simulink library "Aerodynamics_lib"  (R2020a)
settings: Solver=VariableStepAuto  StartTime=0.0  StopTime=10.0  RelTol=1e-3
undefined symbols (not defined in the file or in its folder): bref, CD0, CD_alpha, CL0, Cl_aileron, CL_alpha, CL_alphadot, Cl_beta, CL_elev, Cl_p, CL_q, Cl_r, Cl_rudder, Cm0, Cm_alpha, Cm_alphadot, Cm_elev, Cm_q, Cn_aileron, Cn_beta, Cn_p, Cn_r, Cn_rudder, cref, CY_beta, CY_p, CY_r, CY_rudder, Sref, X_CG, Z_CG
settings Model: Creator=muril  LastModifiedBy=muril

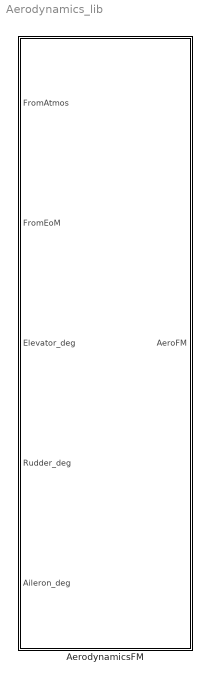
== system Aerodynamics_lib ==
  AerodynamicsFM : Subsystem

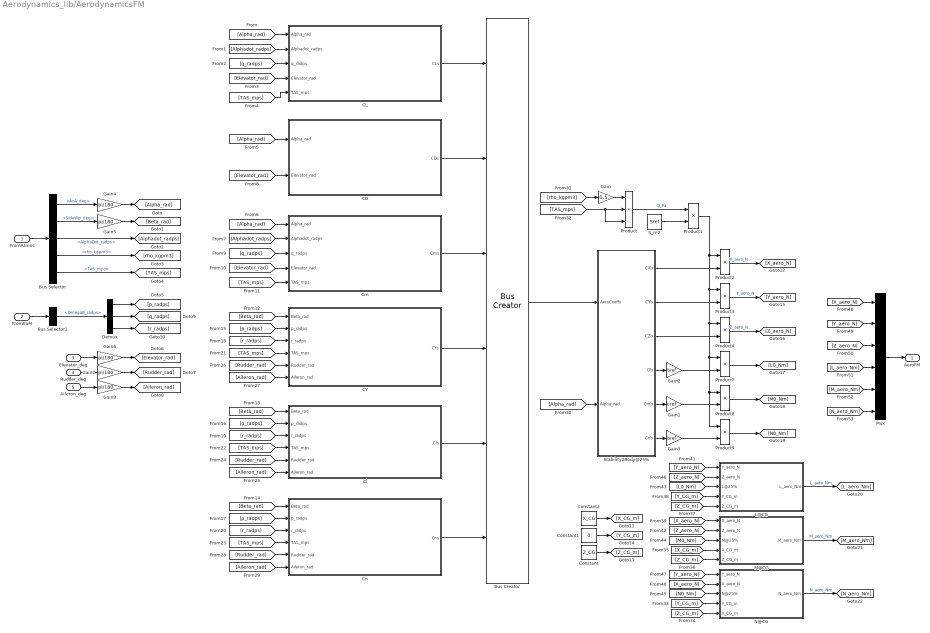
== system Aerodynamics_lib/AerodynamicsFM ==
  FromAtmos : Inport
  FromEoM : Inport  Port=2
  Elevator_deg : Inport  Port=3
  Rudder_deg : Inport  Port=4
  Aileron_deg : Inport  Port=5
  Bus Creator : BusCreator  Inputs=6
  Bus Selector : BusSelector  OutputSignals=AoA_deg,Sideslip_deg,AlphaDot_radps,rho_kgpm3,TAS_mps
  Bus Selector1 : BusSelector  OutputSignals=OmegaB_radps
  CD : Subsystem
  CL : Subsystem
  CY : Subsystem
  Cl : Subsystem
  Cm : Subsystem
  Cn : Subsystem
  Constant : Constant  Value=Z_CG
  Constant1 : Constant  Value=0
  Constant2 : Constant  Value=X_CG
  Demux : Demux  Outputs=3
  Gain : Gain  Gain=0.5
  Gain1 : Gain  Gain=cref
  Gain2 : Gain  Gain=bref
  Gain3 : Gain  Gain=bref
  Gain{4..8} (5 alike) : Gain  Gain=pi/180
  L@CG : Subsystem
  M@CG : Subsystem
  Mux : Mux  Inputs=6
  N@CG : Subsystem
  Product : Product  Inputs=3
  Product{1..4,7..9} (7 alike) : Product
  S_m2 : Constant  Value=Sref
  Stability2Body@25% : Subsystem
  AeroFM : Outport
  wires:
  Constant2/1 -> [X_CG_m]
  Constant/1 -> [Z_CG_m]
  Bus Selector1/1 -> Demux/1  "<OmegaB_radps>"
  FromEoM/1 -> Bus Selector1/1
  Bus Selector/3 -> [Alphadot_radps]  "<AlphaDot_radps>"
  Bus Selector/2 -> Gain5/1  "<Sideslip_deg>"
  Bus Selector/1 -> Gain4/1  "<AoA_deg>"
  FromAtmos/1 -> Bus Selector/1
  [q_radps] -> CL/3(q_radps)
  [Alpha_rad] -> CL/1(Alpha_rad)
  Stability2Body@25%/2(CYb) -> Product3/2
  [Beta_rad] -> Cl/1(Beta_rad)
  Gain8/1 -> [Aileron_rad]
  Elevator_deg/1 -> Gain6/1
  Product1/1 -> Product9/1, Product8/1, Product7/1, Product4/1, Product3/1, Product2/1
  Bus Selector/5 -> [TAS_mps]  "<TAS_mps>"
  Product/1 -> Product1/1  "Q_Pa"
  [Alpha_rad] -> CD/1(Alpha_rad)
  Product8/1 -> [M0_Nm]
  Gain7/1 -> [Rudder_rad]
  Demux/1 -> [p_radps]
  [Alphadot_radps] -> CL/2(Alphadot_radps)
  [r_radps] -> Cl/3(r_radps)
  CD/1(CDs) -> Bus Creator/2
  Aileron_deg/1 -> Gain8/1
  [p_radps] -> Cl/2(p_radps)
  [TAS_mps] -> CL/5(TAS_mps)
  [Alphadot_radps] -> Cm/2(Alphadot_radps)
  [Alpha_rad] -> Cm/1(Alpha_rad)
  [TAS_mps] -> Cm/5(TAS_mps)
  [Beta_rad] -> Cn/1(Beta_rad)
  Gain6/1 -> [Elevator_rad]
  [TAS_mps] -> Product/3, Product/2
  N@CG/1(N_aero_Nm) -> [N_aero_Nm]  "N_aero_Nm"
  [Elevator_rad] -> CD/2(Elevator_rad)
  Gain5/1 -> [Beta_rad]
  Stability2Body@25%/3(CZb) -> Product4/2
  Gain3/1 -> Product9/2
  Product3/1 -> [Y_aero_N]  "Y_aero_N"
  [Aileron_rad] -> Cl/6(Aileron_rad)
  [TAS_mps] -> CY/4(TAS_mps)
  Demux/2 -> [q_radps]
  [TAS_mps] -> Cn/4(TAS_mps)
  [Rudder_rad] -> Cl/5(Rudder_rad)
  [Aileron_rad] -> Cn/6(Aileron_rad)
  [r_radps] -> Cn/3(r_radps)
  CL/1(CLs) -> Bus Creator/1
  [Beta_rad] -> CY/1(Beta_rad)
  [Z_CG_m] -> M@CG/5(Z_CG_m)
  S_m2/1 -> Product1/2
  Stability2Body@25%/4(Clb) -> Gain2/1
  [p_radps] -> CY/2(p_radps)
  Stability2Body@25%/1(CXb) -> Product2/2
  [p_radps] -> Cn/2(p_radps)
  [TAS_mps] -> Cl/4(TAS_mps)
  Gain/1 -> Product/1
  CY/1(CYs) -> Bus Creator/4
  [Rudder_rad] -> Cn/5(Rudder_rad)
  Constant1/1 -> [Y_CG_m]
  Cm/1(Cms) -> Bus Creator/3
  Gain1/1 -> Product8/2
  [Rudder_rad] -> CY/5(Rudder_rad)
  Gain2/1 -> Product7/2
  Cn/1(Cns) -> Bus Creator/6
  [Y_aero_N] -> Mux/2
  Stability2Body@25%/5(Cmb) -> Gain1/1
  [Aileron_rad] -> CY/6(Aileron_rad)
  Rudder_deg/1 -> Gain7/1
  Bus Creator/1 -> Stability2Body@25%/1(AeroCoeffs)
  Product2/1 -> [X_aero_N]  "X_aero_N"
  [X_aero_N] -> M@CG/1(X_aero_N)
  [r_radps] -> CY/3(r_radps)
  [Z_CG_m] -> L@CG/5(Z_CG_m)
  [X_CG_m] -> M@CG/4(X_CG_m)
  [Y_CG_m] -> L@CG/4(Y_CG_m)
  Bus Selector/4 -> [rho_kgpm3]  "<rho_kgpm3>"
  Cl/1(Cls) -> Bus Creator/5
  [q_radps] -> Cm/3(q_radps)
  [Elevator_rad] -> Cm/4(Elevator_rad)
  Product4/1 -> [Z_aero_N]  "Z_aero_N"
  Demux/3 -> [r_radps]
  [Alpha_rad] -> Stability2Body@25%/2(Alpha_rad)
  Product9/1 -> [N0_Nm]
  Gain4/1 -> [Alpha_rad]
  M@CG/1(M_aero_Nm) -> [M_aero_Nm]  "M_aero_Nm"
  [M0_Nm] -> M@CG/3(M@25%)
  [rho_kgpm3] -> Gain/1
  [Z_aero_N] -> L@CG/2(Z_aero_N)
  [Y_aero_N] -> L@CG/1(Y_aero_N)
  [X_aero_N] -> N@CG/2(X_aero_N)
  [Z_CG_m] -> N@CG/5(X_CG_m)
  Product7/1 -> [L0_Nm]
  Mux/1 -> AeroFM/1
  [Z_aero_N] -> Mux/3
  [L0_Nm] -> L@CG/3(L@25%)
  Stability2Body@25%/6(Cnb) -> Gain3/1
  [Y_CG_m] -> N@CG/4(Y_CG_m)
  [N0_Nm] -> N@CG/3(N@25%)
  [Elevator_rad] -> CL/4(Elevator_rad)
  [Y_aero_N] -> N@CG/1(Y_aero_N)
  [L_aero_Nm] -> Mux/4
  [X_aero_N] -> Mux/1
  [Z_aero_N] -> M@CG/2(Z_aero_N)
  [M_aero_Nm] -> Mux/5
  L@CG/1(L_aero_Nm) -> [L_aero_Nm]  "L_aero_Nm"
  [N_aero_Nm] -> Mux/6

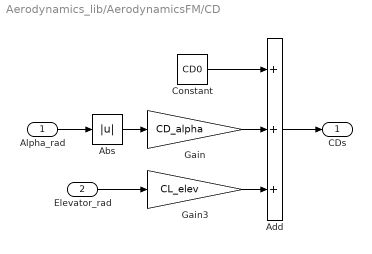
== system Aerodynamics_lib/AerodynamicsFM/CD ==
  Alpha_rad : Inport
  Elevator_rad : Inport  Port=2
  Abs : Abs
  Add : Sum  Inputs=+++
  Constant : Constant  Value=CD0
  Gain : Gain  Gain=CD_alpha
  Gain3 : Gain  Gain=CL_elev
  CDs : Outport
  wires:
  Gain3/1 -> Add/3
  Add/1 -> CDs/1
  Gain/1 -> Add/2
  Constant/1 -> Add/1
  Elevator_rad/1 -> Gain3/1
  Abs/1 -> Gain/1
  Alpha_rad/1 -> Abs/1

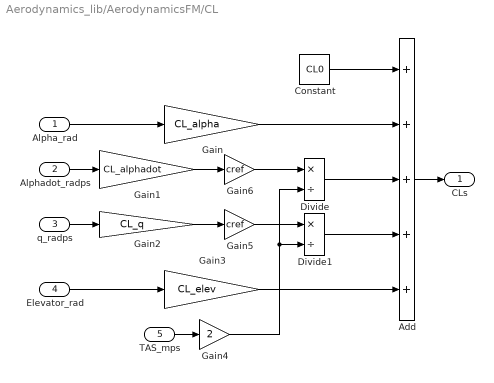
== system Aerodynamics_lib/AerodynamicsFM/CL ==
  Alpha_rad : Inport
  Alphadot_radps : Inport  Port=2
  q_radps : Inport  Port=3
  Elevator_rad : Inport  Port=4
  TAS_mps : Inport  Port=5
  Add : Sum  Inputs=+++++
  Constant : Constant  Value=CL0
  Divide : Product  Inputs=*/
  Divide1 : Product  Inputs=*/
  Gain : Gain  Gain=CL_alpha
  Gain1 : Gain  Gain=CL_alphadot
  Gain2 : Gain  Gain=CL_q
  Gain3 : Gain  Gain=CL_elev
  Gain4 : Gain  Gain=2
  Gain5 : Gain  Gain=cref
  Gain6 : Gain  Gain=cref
  CLs : Outport
  wires:
  Gain3/1 -> Add/5
  Alpha_rad/1 -> Gain/1
  Elevator_rad/1 -> Gain3/1
  Gain/1 -> Add/2
  Alphadot_radps/1 -> Gain1/1
  Constant/1 -> Add/1
  Add/1 -> CLs/1
  TAS_mps/1 -> Gain4/1
  Gain1/1 -> Gain6/1
  Gain6/1 -> Divide/1
  Gain4/1 -> Divide/2, Divide1/2
  Divide/1 -> Add/3
  Divide1/1 -> Add/4
  Gain5/1 -> Divide1/1
  Gain2/1 -> Gain5/1
  q_radps/1 -> Gain2/1

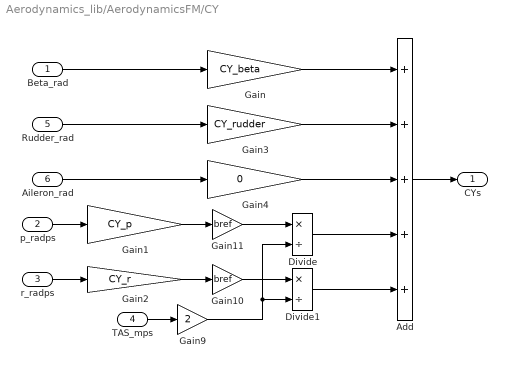
== system Aerodynamics_lib/AerodynamicsFM/CY ==
  Beta_rad : Inport
  p_radps : Inport  Port=2
  r_radps : Inport  Port=3
  TAS_mps : Inport  Port=4
  Rudder_rad : Inport  Port=5
  Aileron_rad : Inport  Port=6
  Add : Sum  Inputs=+++++
  Divide : Product  Inputs=*/
  Divide1 : Product  Inputs=*/
  Gain : Gain  Gain=CY_beta
  Gain1 : Gain  Gain=CY_p
  Gain10 : Gain  Gain=bref
  Gain11 : Gain  Gain=bref
  Gain2 : Gain  Gain=CY_r
  Gain3 : Gain  Gain=CY_rudder
  Gain4 : Gain  Gain=0
  Gain9 : Gain  Gain=2
  CYs : Outport
  wires:
  Gain9/1 -> Divide/2, Divide1/2
  p_radps/1 -> Gain1/1
  Gain1/1 -> Gain11/1
  TAS_mps/1 -> Gain9/1
  Add/1 -> CYs/1
  r_radps/1 -> Gain2/1
  Gain2/1 -> Gain10/1
  Gain10/1 -> Divide1/1
  Beta_rad/1 -> Gain/1
  Gain11/1 -> Divide/1
  Gain/1 -> Add/1
  Divide/1 -> Add/4
  Divide1/1 -> Add/5
  Rudder_rad/1 -> Gain3/1
  Aileron_rad/1 -> Gain4/1
  Gain4/1 -> Add/3
  Gain3/1 -> Add/2

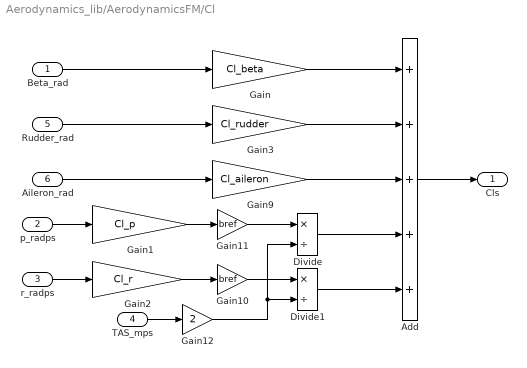
== system Aerodynamics_lib/AerodynamicsFM/Cl ==
  Beta_rad : Inport
  p_radps : Inport  Port=2
  r_radps : Inport  Port=3
  TAS_mps : Inport  Port=4
  Rudder_rad : Inport  Port=5
  Aileron_rad : Inport  Port=6
  Add : Sum  Inputs=+++++
  Divide : Product  Inputs=*/
  Divide1 : Product  Inputs=*/
  Gain : Gain  Gain=Cl_beta
  Gain1 : Gain  Gain=Cl_p
  Gain10 : Gain  Gain=bref
  Gain11 : Gain  Gain=bref
  Gain12 : Gain  Gain=2
  Gain2 : Gain  Gain=Cl_r
  Gain3 : Gain  Gain=Cl_rudder
  Gain9 : Gain  Gain=Cl_aileron
  Cls : Outport
  wires:
  r_radps/1 -> Gain2/1
  Gain12/1 -> Divide/2, Divide1/2
  Divide/1 -> Add/4
  Gain1/1 -> Gain11/1
  Gain/1 -> Add/1
  Aileron_rad/1 -> Gain9/1
  Gain10/1 -> Divide1/1
  p_radps/1 -> Gain1/1
  Divide1/1 -> Add/5
  Add/1 -> Cls/1
  TAS_mps/1 -> Gain12/1
  Gain2/1 -> Gain10/1
  Gain11/1 -> Divide/1
  Rudder_rad/1 -> Gain3/1
  Beta_rad/1 -> Gain/1
  Gain9/1 -> Add/3
  Gain3/1 -> Add/2

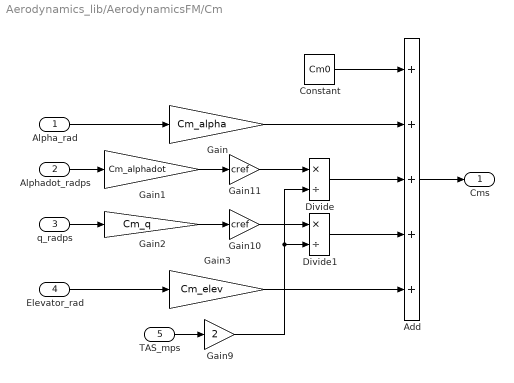
== system Aerodynamics_lib/AerodynamicsFM/Cm ==
  Alpha_rad : Inport
  Alphadot_radps : Inport  Port=2
  q_radps : Inport  Port=3
  Elevator_rad : Inport  Port=4
  TAS_mps : Inport  Port=5
  Add : Sum  Inputs=+++++
  Constant : Constant  Value=Cm0
  Divide : Product  Inputs=*/
  Divide1 : Product  Inputs=*/
  Gain : Gain  Gain=Cm_alpha
  Gain1 : Gain  Gain=Cm_alphadot
  Gain10 : Gain  Gain=cref
  Gain11 : Gain  Gain=cref
  Gain2 : Gain  Gain=Cm_q
  Gain3 : Gain  Gain=Cm_elev
  Gain9 : Gain  Gain=2
  Cms : Outport
  wires:
  Gain2/1 -> Gain10/1
  Gain/1 -> Add/2
  Gain11/1 -> Divide/1
  Gain9/1 -> Divide/2, Divide1/2
  TAS_mps/1 -> Gain9/1
  Constant/1 -> Add/1
  Divide1/1 -> Add/4
  q_radps/1 -> Gain2/1
  Gain3/1 -> Add/5
  Elevator_rad/1 -> Gain3/1
  Gain1/1 -> Gain11/1
  Alphadot_radps/1 -> Gain1/1
  Gain10/1 -> Divide1/1
  Divide/1 -> Add/3
  Alpha_rad/1 -> Gain/1
  Add/1 -> Cms/1

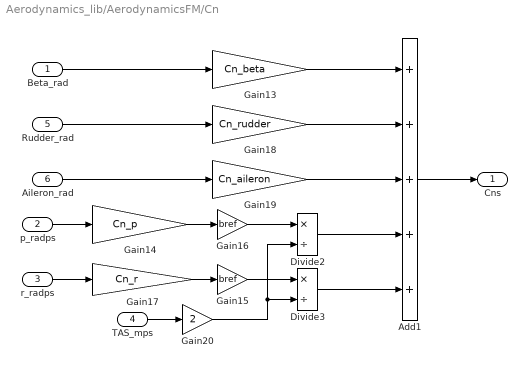
== system Aerodynamics_lib/AerodynamicsFM/Cn ==
  Beta_rad : Inport
  p_radps : Inport  Port=2
  r_radps : Inport  Port=3
  TAS_mps : Inport  Port=4
  Rudder_rad : Inport  Port=5
  Aileron_rad : Inport  Port=6
  Add1 : Sum  Inputs=+++++
  Divide2 : Product  Inputs=*/
  Divide3 : Product  Inputs=*/
  Gain13 : Gain  Gain=Cn_beta
  Gain14 : Gain  Gain=Cn_p
  Gain15 : Gain  Gain=bref
  Gain16 : Gain  Gain=bref
  Gain17 : Gain  Gain=Cn_r
  Gain18 : Gain  Gain=Cn_rudder
  Gain19 : Gain  Gain=Cn_aileron
  Gain20 : Gain  Gain=2
  Cns : Outport
  wires:
  Beta_rad/1 -> Gain13/1
  Gain20/1 -> Divide2/2, Divide3/2
  Divide2/1 -> Add1/4
  Divide3/1 -> Add1/5
  Aileron_rad/1 -> Gain19/1
  Gain14/1 -> Gain16/1
  TAS_mps/1 -> Gain20/1
  Gain13/1 -> Add1/1
  r_radps/1 -> Gain17/1
  Gain17/1 -> Gain15/1
  Add1/1 -> Cns/1
  Gain16/1 -> Divide2/1
  Gain15/1 -> Divide3/1
  Rudder_rad/1 -> Gain18/1
  p_radps/1 -> Gain14/1
  Gain19/1 -> Add1/3
  Gain18/1 -> Add1/2

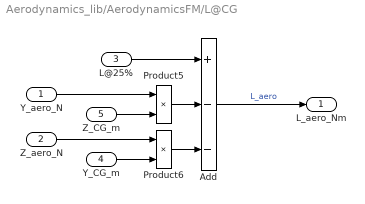
== system Aerodynamics_lib/AerodynamicsFM/L@CG ==
  Y_aero_N : Inport
  Z_aero_N : Inport  Port=2
  L@25% : Inport  Port=3
  Y_CG_m : Inport  Port=4
  Z_CG_m : Inport  Port=5
  Add : Sum  Inputs=+--
  Product5 : Product
  Product6 : Product
  L_aero_Nm : Outport
  wires:
  Product6/1 -> Add/3
  Z_aero_N/1 -> Product6/1
  Z_CG_m/1 -> Product5/2
  Product5/1 -> Add/2
  Y_aero_N/1 -> Product5/1
  Add/1 -> L_aero_Nm/1  "L_aero"
  L@25%/1 -> Add/1
  Y_CG_m/1 -> Product6/2

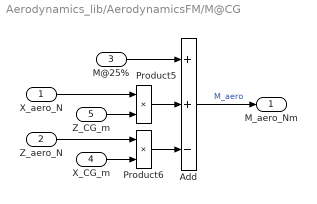
== system Aerodynamics_lib/AerodynamicsFM/M@CG ==
  X_aero_N : Inport
  Z_aero_N : Inport  Port=2
  M@25% : Inport  Port=3
  X_CG_m : Inport  Port=4
  Z_CG_m : Inport  Port=5
  Add : Sum  Inputs=++-
  Product5 : Product
  Product6 : Product
  M_aero_Nm : Outport
  wires:
  Add/1 -> M_aero_Nm/1  "M_aero"
  Z_aero_N/1 -> Product6/1
  Product6/1 -> Add/3
  X_CG_m/1 -> Product6/2
  X_aero_N/1 -> Product5/1
  Product5/1 -> Add/2
  Z_CG_m/1 -> Product5/2
  M@25%/1 -> Add/1

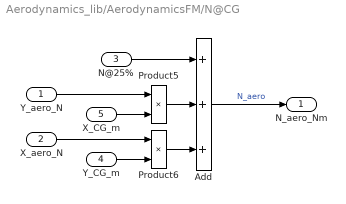
== system Aerodynamics_lib/AerodynamicsFM/N@CG ==
  Y_aero_N : Inport
  X_aero_N : Inport  Port=2
  N@25% : Inport  Port=3
  Y_CG_m : Inport  Port=4
  X_CG_m : Inport  Port=5
  Add : Sum  Inputs=+++
  Product5 : Product
  Product6 : Product
  N_aero_Nm : Outport
  wires:
  Y_CG_m/1 -> Product6/2
  Product5/1 -> Add/2
  N@25%/1 -> Add/1
  Product6/1 -> Add/3
  Add/1 -> N_aero_Nm/1  "N_aero"
  X_CG_m/1 -> Product5/2
  Y_aero_N/1 -> Product5/1
  X_aero_N/1 -> Product6/1

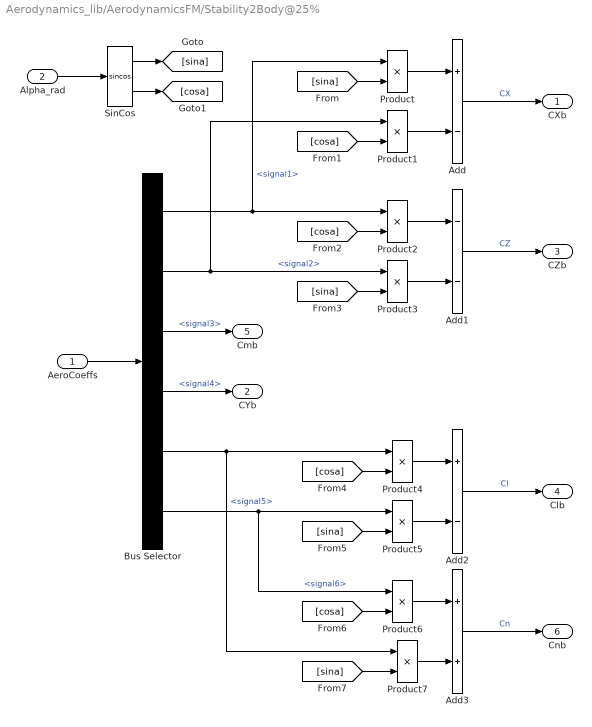
== system Aerodynamics_lib/AerodynamicsFM/Stability2Body@25% ==
  AeroCoeffs : Inport
  Alpha_rad : Inport  Port=2
  Add : Sum  Inputs=+-
  Add1 : Sum  Inputs=--
  Add2 : Sum  Inputs=+-
  Add3 : Sum
  Bus Selector : BusSelector  OutputSignals=signal1,signal2,signal3,signal4,signal5,signal6
  Product{,1..7} (8 alike) : Product
  SinCos : Trigonometry  Operator=sincos
  CXb : Outport
  CYb : Outport  Port=2
  CZb : Outport  Port=3
  Clb : Outport  Port=4
  Cmb : Outport  Port=5
  Cnb : Outport  Port=6
  wires:
  AeroCoeffs/1 -> Bus Selector/1
  Alpha_rad/1 -> SinCos/1
  SinCos/1 -> [sina]
  SinCos/2 -> [cosa]
  [sina] -> Product/2
  [cosa] -> Product1/2
  Product/1 -> Add/1
  Product1/1 -> Add/2
  Add/1 -> CXb/1  "CX"
  Product3/1 -> Add1/2
  Bus Selector/1 -> Product2/1, Product/1  "<signal1>"
  [cosa] -> Product2/2
  Product2/1 -> Add1/1
  [sina] -> Product3/2
  Bus Selector/2 -> Product3/1, Product1/1  "<signal2>"
  Add1/1 -> CZb/1  "CZ"
  [cosa] -> Product4/2
  Bus Selector/5 -> Product7/1, Product4/1  "<signal5>"
  [sina] -> Product5/2
  Bus Selector/6 -> Product6/1, Product5/1  "<signal6>"
  Product4/1 -> Add2/1
  Product5/1 -> Add2/2
  Add2/1 -> Clb/1  "Cl"
  [cosa] -> Product6/2
  [sina] -> Product7/2
  Product6/1 -> Add3/1
  Product7/1 -> Add3/2
  Add3/1 -> Cnb/1  "Cn"
  Bus Selector/4 -> CYb/1  "<signal4>"
  Bus Selector/3 -> Cmb/1  "<signal3>"
